simulink model "SimpleStack"  (R2023b)
settings: Solver=ode4  StartTime=0.0  StopTime=10.0  FixedStep=1e-4  RelTol=1e-6
undefined symbols (not defined in the file): A_stack, M_H2O, M_Nmix, M_O2, m_st_Nmix_init, m_st_O2_init, m_st_vp_init, R_Nmix, R_O2, R_vp, V_stack
settings Model: Creator=KOTA-Z  LastModifiedBy=KOTA-Z

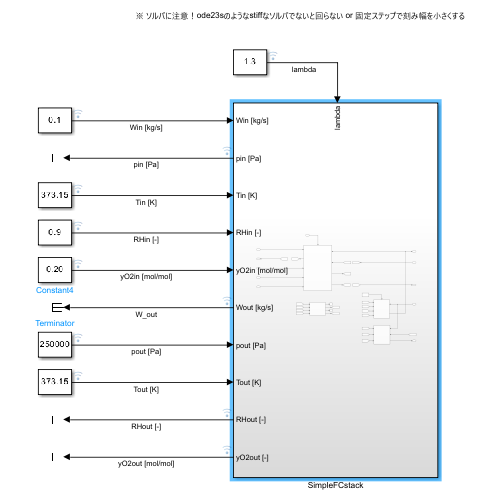
[thumbnail: Simulink's stored preview of the top-level diagram]
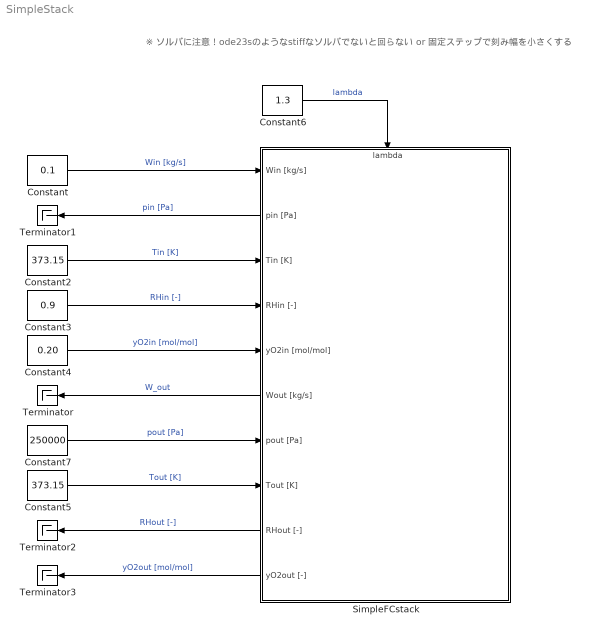
== system SimpleStack ==
  note: ※ ソルバに注意！ode23sのようなstiffなソルバでないと回らない or 固定ステップで刻み幅を小さくする
  Constant : Constant  Value=0.1
  Constant2 : Constant  Value=373.15
  Constant3 : Constant  Value=0.9
  Constant4 : Constant  Value=0.20
  Constant5 : Constant  Value=373.15
  Constant6 : Constant  Value=1.3
  Constant7 : Constant  Value=250000
  SimpleFCstack : Subsystem
      settings: PortSchema="{\"entries\":[{\"content\":{\"sides\":[{\"content\":{\"connectorIds\":[\"In1\",\"Out1\",\"In2\",\"In3\",\"In4\",\"Out2\",\"In5\",\"In6\",\"Out3\",\"Out4\"]},\"type\":\"ConnectorPlacement.EquallySpacedRectSide\",\"uuid\":\"655c3a5c-2438-4b8a-8343-42ad601375b4\"},{\"content\":{\"side\":\"RIGHT\"},\"type\":\"ConnectorPlacement.EquallySpacedRectSide\",\"uuid\":\"d33e9b8c-45a6-4977-af4d-86fbf3e4639a\"},{\"content\":{\"connectorIds\":[\"In7\"],\"side\":\"TOP\"},\"type\":\"ConnectorPlacement.EquallySpacedRectSide\",\"uuid\":\"600fa4b4-34fc-436b-99fc-6adfd4c4a471\"}]},\"type\":\"ConnectorPlacement.EquallySpacedConnector\",\"uuid\":\"963465b0-aa19-4ba1-823c-60c91f5f4c3b\"}],\"packageUris\":[\"http://schema.mathworks.com/mf0/Connector/R2020b\"],\"version\":\"1.0\"}"
  Terminator{,1..3} (4 alike) : Terminator
  wires:
  Constant5/1 -> SimpleFCstack/6(Tout [K])  "Tout [K]"
  Constant4/1 -> SimpleFCstack/4(yO2in [mol/mol])  "yO2in [mol/mol]"
  Constant/1 -> SimpleFCstack/1(Win [kg/s])  "Win [kg/s]"
  Constant3/1 -> SimpleFCstack/3(RHin [-])  "RHin [-]"
  SimpleFCstack/1(pin [Pa]) -> Terminator1/1  "pin [Pa]"
  SimpleFCstack/4(yO2out [-]) -> Terminator3/1  "yO2out [mol/mol]"
  Constant7/1 -> SimpleFCstack/5(pout [Pa])  "pout [Pa]"
  SimpleFCstack/2(Wout [kg/s]) -> Terminator/1  "W_out"
  Constant6/1 -> SimpleFCstack/7(lambda)  "lambda"
  SimpleFCstack/3(RHout [-]) -> Terminator2/1  "RHout [-]"
  Constant2/1 -> SimpleFCstack/2(Tin [K])  "Tin [K]"

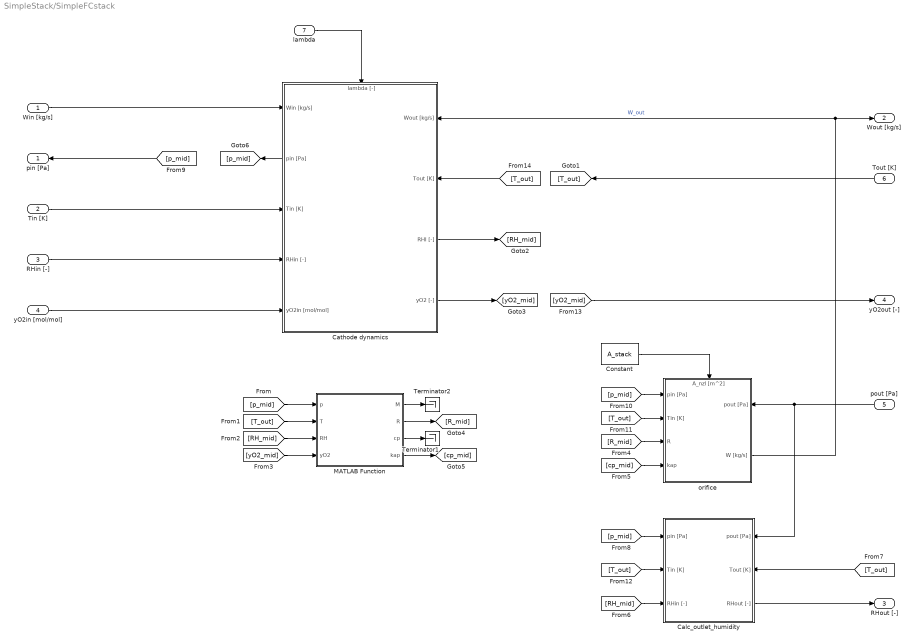
== system SimpleStack/SimpleFCstack ==
  Win [kg/s] : Inport
  Tin [K] : Inport  Port=2
  RHin [-] : Inport  Port=3
  yO2in [mol/mol] : Inport  Port=4
  pout [Pa] : Inport  Port=5
  Tout [K] : Inport  Port=6
  lambda : Inport  Port=7
  Calc_outlet_humidity : Subsystem
      settings: PortSchema="{\"entries\":[{\"content\":{\"sides\":[{\"content\":{\"connectorIds\":[\"In1\",\"In2\",\"In3\"]},\"type\":\"ConnectorPlacement.EquallySpacedRectSide\",\"uuid\":\"71f38106-807e-4ed0-ae6c-bbacb474f6c2\"},{\"content\":{\"connectorIds\":[\"In4\",\"In5\",\"Out1\"],\"side\":\"RIGHT\"},\"type\":\"ConnectorPlacement.EquallySpacedRectSide\",\"uuid\":\"6d4269b2-3333-4431-9298-369e5f90d9a7\"},{\"content\":{\"side\":\"TOP\"},\"type\":\"ConnectorPlacement.EquallySpacedRectSide\",\"uuid\":\"5a9c4429-cecf-425a-a491-b651e9aa4143\"}]},\"type\":\"ConnectorPlacement.EquallySpacedConnector\",\"uuid\":\"39426d6a-7e43-41a2-9c81-324c7c3acccd\"}],\"packageUris\":[\"http://schema.mathworks.com/mf0/Connector/R2020b\"],\"version\":\"1.0\"}"
  Cathode dynamics : Subsystem
      settings: PortSchema="{\"entries\":[{\"content\":{\"sides\":[{\"content\":{\"connectorIds\":[\"In1\",\"Out3\",\"In2\",\"In3\",\"In4\"]},\"type\":\"ConnectorPlacement.EquallySpacedRectSide\",\"uuid\":\"fa7fb944-b3f2-4d7f-acb3-ff4b9695f5bb\"},{\"content\":{\"connectorIds\":[\"In6\",\"In7\",\"Out1\",\"Out2\"],\"side\":\"RIGHT\"},\"type\":\"ConnectorPlacement.EquallySpacedRectSide\",\"uuid\":\"c44f1f17-fb15-4535-ad6a-0eca26be82eb\"},{\"content\":{\"connectorIds\":[\"In5\"],\"side\":\"TOP\"},\"type\":\"ConnectorPlacement.EquallySpacedRectSide\",\"uuid\":\"3976ae6f-6c41-45df-9f2a-11517639fca1\"}]},\"type\":\"ConnectorPlacement.EquallySpacedConnector\",\"uuid\":\"2e8d1e31-2d62-44f7-94c0-4e740688e650\"}],\"packageUris\":[\"http://schema.mathworks.com/mf0/Connector/R2020b\"],\"version\":\"1.0\"}"
  Constant : Constant  Value=A_stack
  MATLAB Function : MATLAB Function  TreatAsAtomicUnit=on  mask{M_O2=M_O2, M_Nmix=M_Nmix, M_H2O=M_H2O}
      mask prompts: M_O2 "Molar mass O2 [kg/mol]"; M_Nmix "Molar mass Nmix [kg/mol]"; M_H2O "Molar mass H2O [kg/mol]"
  Terminator1 : Terminator
  Terminator2 : Terminator
  orifice : Subsystem
      settings: PortSchema="{\"entries\":[{\"content\":{\"sides\":[{\"content\":{\"connectorIds\":[\"In1\",\"In2\",\"In3\",\"In4\"]},\"type\":\"ConnectorPlacement.EquallySpacedRectSide\",\"uuid\":\"efae8970-47c5-4a02-bf2c-57821bb85d37\"},{\"content\":{\"connectorIds\":[\"In6\",\"Out1\"],\"side\":\"RIGHT\"},\"type\":\"ConnectorPlacement.EquallySpacedRectSide\",\"uuid\":\"c072edf9-8db2-4656-9a6c-525b54cf676d\"},{\"content\":{\"connectorIds\":[\"In5\"],\"side\":\"TOP\"},\"type\":\"ConnectorPlacement.EquallySpacedRectSide\",\"uuid\":\"a5f35e53-894b-4e4e-8f09-bf3a2c067244\"},{\"content\":{\"side\":\"BOTTOM\"},\"type\":\"ConnectorPlacement.EquallySpacedRectSide\",\"uuid\":\"c3ea8794-d4c2-446d-854c-4c5a5875e6e6\"}]},\"type\":\"ConnectorPlacement.EquallySpacedConnector\",\"uuid\":\"567c8408-e503-409c-8be3-b925cf408148\"}],\"packageUris\":[\"http://schema.mathworks.com/mf0/Connector/R2020b\"],\"version\":\"1.0\"}"
  pin [Pa] : Outport
  Wout [kg/s] : Outport  Port=2
  RHout [-] : Outport  Port=3
  yO2out [-] : Outport  Port=4
  wires:
  pout [Pa]/1 -> orifice/6(pout [Pa]), Calc_outlet_humidity/4(pout [Pa])
  orifice/1(W [kg/s]) -> Cathode dynamics/6(Wout [kg/s]), Wout [kg/s]/1  "W_out"
  Constant/1 -> orifice/5(A_nzl [m^2])
  Cathode dynamics/2(yO2 [-]) -> [yO2_mid]
  Win [kg/s]/1 -> Cathode dynamics/1(Win [kg/s])
  [p_mid] -> pin [Pa]/1
  lambda/1 -> Cathode dynamics/5(lambda [-])
  Tin [K]/1 -> Cathode dynamics/2(Tin [K])
  RHin [-]/1 -> Cathode dynamics/3(RHin [-])
  yO2in [mol/mol]/1 -> Cathode dynamics/4(yO2in [mol/mol])
  Calc_outlet_humidity/1(RHout [-]) -> RHout [-]/1
  MATLAB Function/1(M) -> Terminator2/1
  MATLAB Function/3(cp) -> Terminator1/1
  Cathode dynamics/1(RHI [-]) -> [RH_mid]
  [p_mid] -> MATLAB Function/1(p)
  [T_out] -> MATLAB Function/2(T)
  [RH_mid] -> MATLAB Function/3(RH)
  [yO2_mid] -> MATLAB Function/4(yO2)
  MATLAB Function/2(R) -> [R_mid]
  [R_mid] -> orifice/3(R)
  MATLAB Function/4(kap) -> [cp_mid]
  [cp_mid] -> orifice/4(kap)
  [RH_mid] -> Calc_outlet_humidity/3(RHin [-])
  [T_out] -> Calc_outlet_humidity/5(Tout [K])
  [p_mid] -> Calc_outlet_humidity/1(pin [Pa])
  Cathode dynamics/3(pin [Pa]) -> [p_mid]
  [p_mid] -> orifice/1(pin [Pa])
  [T_out] -> orifice/2(Tin [K])
  [T_out] -> Calc_outlet_humidity/2(Tin [K])
  [yO2_mid] -> yO2out [-]/1
  [T_out] -> Cathode dynamics/7(Tout [K])
  Tout [K]/1 -> [T_out]

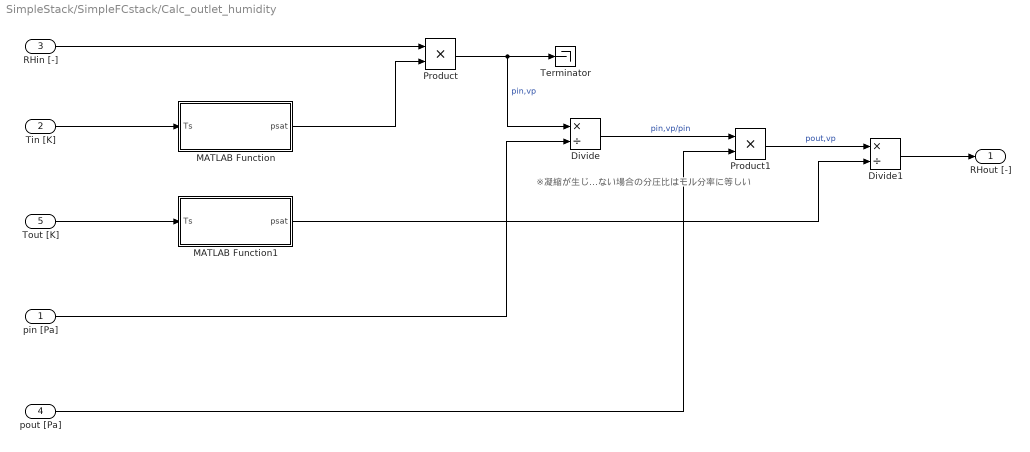
== system SimpleStack/SimpleFCstack/Calc_outlet_humidity ==
  note: ※凝縮が生じない場合の分圧比はモル分率に等しい
  pin [Pa] : Inport
  Tin [K] : Inport  Port=2
  RHin [-] : Inport  Port=3
  pout [Pa] : Inport  Port=4
  Tout [K] : Inport  Port=5
  Divide : Product  Inputs=*/
  Divide1 : Product  Inputs=*/
  MATLAB Function : MATLAB Function  TreatAsAtomicUnit=on
  MATLAB Function1 : MATLAB Function  TreatAsAtomicUnit=on
  Product : Product
  Product1 : Product
  Terminator : Terminator
  RHout [-] : Outport
  wires:
  MATLAB Function/1(psat) -> Product/2
  Tin [K]/1 -> MATLAB Function/1(Ts)
  Tout [K]/1 -> MATLAB Function1/1(Ts)
  RHin [-]/1 -> Product/1
  Product/1 -> Terminator/1, Divide/1  "pin,vp"
  pin [Pa]/1 -> Divide/2
  Divide/1 -> Product1/1  "pin,vp/pin"
  pout [Pa]/1 -> Product1/2
  Product1/1 -> Divide1/1  "pout,vp"
  MATLAB Function1/1(psat) -> Divide1/2
  Divide1/1 -> RHout [-]/1

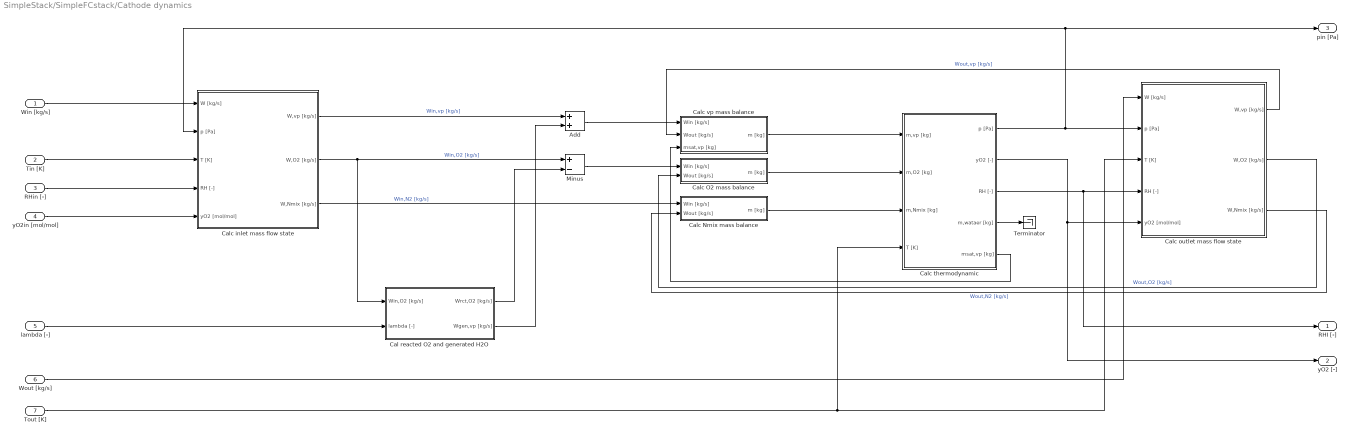
== system SimpleStack/SimpleFCstack/Cathode dynamics ==
  Win [kg/s] : Inport
  Tin [K] : Inport  Port=2
  RHin [-] : Inport  Port=3
  yO2in [mol/mol] : Inport  Port=4
  lambda [-] : Inport  Port=5
  Wout [kg/s] : Inport  Port=6
  Tout [K] : Inport  Port=7
  Add : Sum
  Cal reacted O2 and generated H2O : Subsystem
  Calc Nmix mass balance : Subsystem
  Calc O2 mass balance : Subsystem
  Calc inlet mass flow state : Subsystem
  Calc outlet mass flow state : Subsystem
  Calc thermodynamic : Subsystem
  Calc vp mass balance : Subsystem
  Minus : Sum  Inputs=+-
  Terminator : Terminator
  RHI [-] : Outport
  yO2 [-] : Outport  Port=2
  pin [Pa] : Outport  Port=3
  wires:
  Calc outlet mass flow state/3(W,Nmix [kg/s]) -> Calc Nmix mass balance/2(Wout [kg/s])  "Wout,N2 [kg/s]"
  Calc vp mass balance/1(m [kg]) -> Calc thermodynamic/1(m,vp [kg])
  RHin [-]/1 -> Calc inlet mass flow state/4(RH [-])
  Calc outlet mass flow state/1(W,vp [kg/s]) -> Calc vp mass balance/2(Wout [kg/s])  "Wout,vp [kg/s]"
  Calc inlet mass flow state/2(W,O2 [kg/s]) -> Minus/1, Cal reacted O2 and generated H2O/1(Win,O2 [kg/s])  "Win,O2 [kg/s]"
  Win [kg/s]/1 -> Calc inlet mass flow state/1(W [kg/s])
  Calc O2 mass balance/1(m [kg]) -> Calc thermodynamic/2(m,O2 [kg])
  lambda [-]/1 -> Cal reacted O2 and generated H2O/2(lambda [-])
  Minus/1 -> Calc O2 mass balance/1(Win [kg/s])
  Calc thermodynamic/2(yO2 [-]) -> yO2 [-]/1, Calc outlet mass flow state/5(yO2 [mol/mol])
  Tout [K]/1 -> Calc outlet mass flow state/3(T [K]), Calc thermodynamic/4(T [K])
  Calc outlet mass flow state/2(W,O2 [kg/s]) -> Calc O2 mass balance/2(Wout [kg/s])  "Wout,O2 [kg/s]"
  Calc inlet mass flow state/3(W,Nmix [kg/s]) -> Calc Nmix mass balance/1(Win [kg/s])  "Win,N2 [kg/s]"
  Calc Nmix mass balance/1(m [kg]) -> Calc thermodynamic/3(m,Nmix [kg])
  Calc thermodynamic/3(RH [-]) -> RHI [-]/1, Calc outlet mass flow state/4(RH [-])
  Calc thermodynamic/4(m,wataer [kg]) -> Terminator/1
  Cal reacted O2 and generated H2O/1(Wrct,O2 [kg/s]) -> Minus/2
  Calc thermodynamic/5(msat,vp [kg]) -> Calc vp mass balance/3(msat,vp [kg])
  Tin [K]/1 -> Calc inlet mass flow state/3(T [K])
  Calc inlet mass flow state/1(W,vp [kg/s]) -> Add/1  "Win,vp [kg/s]"
  Add/1 -> Calc vp mass balance/1(Win [kg/s])
  yO2in [mol/mol]/1 -> Calc inlet mass flow state/5(yO2 [mol/mol])
  Cal reacted O2 and generated H2O/2(Wgen,vp [kg/s]) -> Add/2
  Calc thermodynamic/1(p [Pa]) -> pin [Pa]/1, Calc inlet mass flow state/2(p [Pa]), Calc outlet mass flow state/2(p [Pa])
  Wout [kg/s]/1 -> Calc outlet mass flow state/1(W [kg/s])

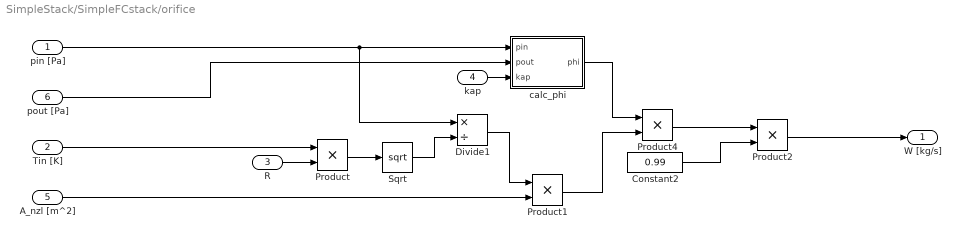
== system SimpleStack/SimpleFCstack/orifice ==
  pin [Pa] : Inport
  Tin [K] : Inport  Port=2
  R : Inport  Port=3
  kap : Inport  Port=4
  A_nzl [m^2] : Inport  Port=5
  pout [Pa] : Inport  Port=6
  Constant2 : Constant  Value=0.99
  Divide1 : Product  Inputs=*/
  Product{,1..2,4} (4 alike) : Product
  Sqrt : Sqrt
  calc_phi : MATLAB Function  TreatAsAtomicUnit=on
  W [kg/s] : Outport
  wires:
  pout [Pa]/1 -> calc_phi/2(pout)
  pin [Pa]/1 -> calc_phi/1(pin), Divide1/1
  Tin [K]/1 -> Product/1
  A_nzl [m^2]/1 -> Product1/2
  R/1 -> Product/2
  Product/1 -> Sqrt/1
  Sqrt/1 -> Divide1/2
  Divide1/1 -> Product1/1
  kap/1 -> calc_phi/3(kap)
  calc_phi/1(phi) -> Product4/1
  Product1/1 -> Product4/2
  Product4/1 -> Product2/1
  Product2/1 -> W [kg/s]/1
  Constant2/1 -> Product2/2

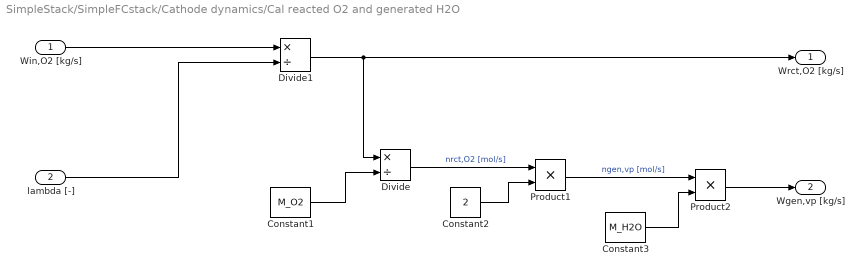
== system SimpleStack/SimpleFCstack/Cathode dynamics/Cal reacted O2 and generated H2O ==
  Win,O2 [kg/s] : Inport
  lambda [-] : Inport  Port=2
  Constant1 : Constant  Value=M_O2
  Constant2 : Constant  Value=2
  Constant3 : Constant  Value=M_H2O
  Divide : Product  Inputs=*/
  Divide1 : Product  Inputs=*/  RndMeth=Zero  SaturateOnIntegerOverflow=on
  Product1 : Product
  Product2 : Product
  Wrct,O2 [kg/s] : Outport
  Wgen,vp [kg/s] : Outport  Port=2
  wires:
  Divide1/1 -> Wrct,O2 [kg/s]/1, Divide/1
  Win,O2 [kg/s]/1 -> Divide1/1
  Constant1/1 -> Divide/2
  Divide/1 -> Product1/1  "nrct,O2 [mol/s]"
  Constant2/1 -> Product1/2
  Product1/1 -> Product2/1  "ngen,vp [mol/s]"
  Constant3/1 -> Product2/2
  Product2/1 -> Wgen,vp [kg/s]/1
  lambda [-]/1 -> Divide1/2

== system SimpleStack/SimpleFCstack/Cathode dynamics/Calc Nmix mass balance ==
  Win [kg/s] : Inport
  Wout [kg/s] : Inport  Port=2
  Integrator : Integrator  InitialCondition=m_st_Nmix_init
  Minus : Sum  Inputs=+-
  m [kg] : Outport
  wires:
  Win [kg/s]/1 -> Minus/1
  Wout [kg/s]/1 -> Minus/2
  Minus/1 -> Integrator/1
  Integrator/1 -> m [kg]/1

== system SimpleStack/SimpleFCstack/Cathode dynamics/Calc O2 mass balance ==
  Win [kg/s] : Inport
  Wout [kg/s] : Inport  Port=2
  Integrator : Integrator  InitialCondition=m_st_O2_init
  Minus : Sum  Inputs=+-
  m [kg] : Outport
  wires:
  Integrator/1 -> m [kg]/1
  Minus/1 -> Integrator/1
  Wout [kg/s]/1 -> Minus/2
  Win [kg/s]/1 -> Minus/1

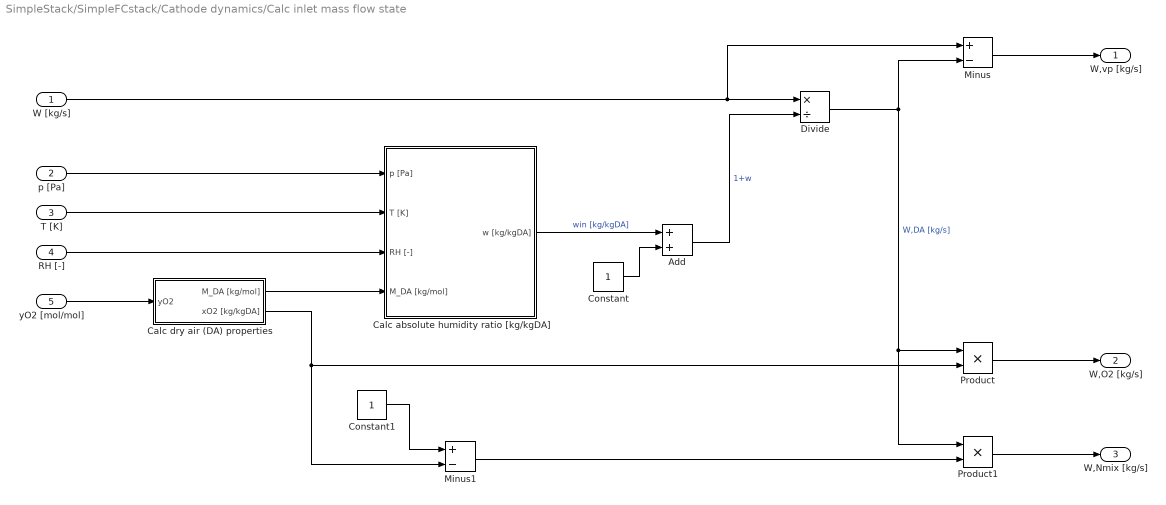
== system SimpleStack/SimpleFCstack/Cathode dynamics/Calc inlet mass flow state ==
  W [kg/s] : Inport
  p [Pa] : Inport  Port=2
  T [K] : Inport  Port=3
  RH [-] : Inport  Port=4
  yO2 [mol/mol] : Inport  Port=5
  Add : Sum
  Calc absolute humidity ratio [kg/kgDA] : Subsystem
  Calc dry air (DA) properties : Subsystem
  Constant : Constant
  Constant1 : Constant
  Divide : Product  Inputs=*/
  Minus : Sum  Inputs=+-
  Minus1 : Sum  Inputs=+-
  Product : Product
  Product1 : Product
  W,vp [kg/s] : Outport
  W,O2 [kg/s] : Outport  Port=2
  W,Nmix [kg/s] : Outport  Port=3
  wires:
  p [Pa]/1 -> Calc absolute humidity ratio [kg/kgDA]/1(p [Pa])
  Calc dry air (DA) properties/2(xO2 [kg/kgDA]) -> Minus1/2, Product/2
  Calc absolute humidity ratio [kg/kgDA]/1(w [kg/kgDA]) -> Add/1  "win [kg/kgDA]"
  Calc dry air (DA) properties/1(M_DA [kg/mol]) -> Calc absolute humidity ratio [kg/kgDA]/4(M_DA [kg/mol])
  Product/1 -> W,O2 [kg/s]/1
  Divide/1 -> Minus/2, Product1/1, Product/1  "W,DA [kg/s]"
  Product1/1 -> W,Nmix [kg/s]/1
  Minus1/1 -> Product1/2
  Minus/1 -> W,vp [kg/s]/1
  yO2 [mol/mol]/1 -> Calc dry air (DA) properties/1(yO2)
  Constant1/1 -> Minus1/1
  RH [-]/1 -> Calc absolute humidity ratio [kg/kgDA]/3(RH [-])
  W [kg/s]/1 -> Minus/1, Divide/1
  Constant/1 -> Add/2
  Add/1 -> Divide/2  "1+w"
  T [K]/1 -> Calc absolute humidity ratio [kg/kgDA]/2(T [K])

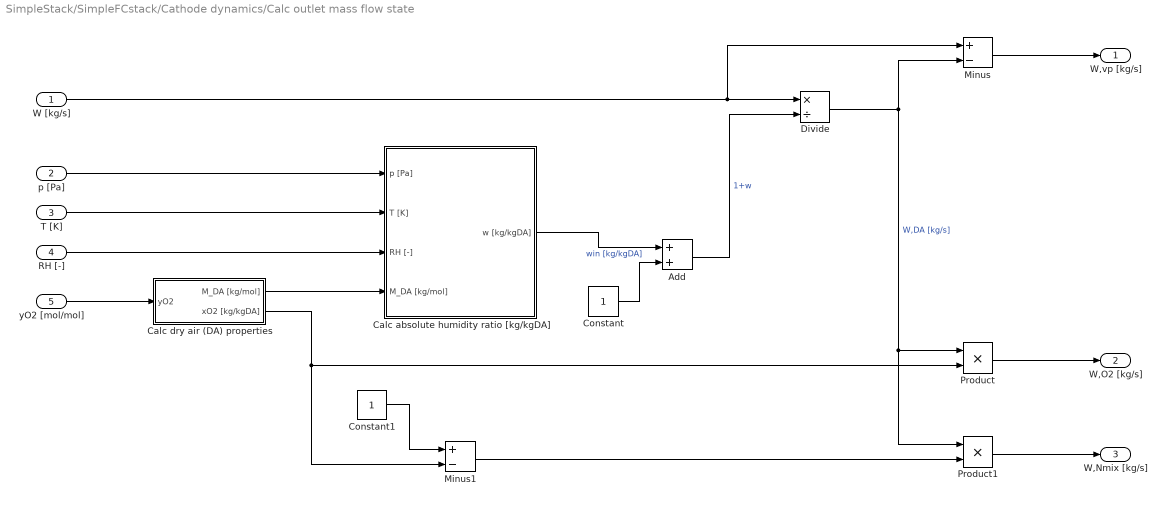
== system SimpleStack/SimpleFCstack/Cathode dynamics/Calc outlet mass flow state ==
  W [kg/s] : Inport
  p [Pa] : Inport  Port=2
  T [K] : Inport  Port=3
  RH [-] : Inport  Port=4
  yO2 [mol/mol] : Inport  Port=5
  Add : Sum
  Calc absolute humidity ratio [kg/kgDA] : Subsystem
  Calc dry air (DA) properties : Subsystem
  Constant : Constant
  Constant1 : Constant
  Divide : Product  Inputs=*/
  Minus : Sum  Inputs=+-
  Minus1 : Sum  Inputs=+-
  Product : Product
  Product1 : Product
  W,vp [kg/s] : Outport
  W,O2 [kg/s] : Outport  Port=2
  W,Nmix [kg/s] : Outport  Port=3
  wires:
  T [K]/1 -> Calc absolute humidity ratio [kg/kgDA]/2(T [K])
  Add/1 -> Divide/2  "1+w"
  Constant/1 -> Add/2
  W [kg/s]/1 -> Divide/1, Minus/1
  RH [-]/1 -> Calc absolute humidity ratio [kg/kgDA]/3(RH [-])
  Constant1/1 -> Minus1/1
  yO2 [mol/mol]/1 -> Calc dry air (DA) properties/1(yO2)
  Minus/1 -> W,vp [kg/s]/1
  Minus1/1 -> Product1/2
  Product1/1 -> W,Nmix [kg/s]/1
  Divide/1 -> Product/1, Product1/1, Minus/2  "W,DA [kg/s]"
  Product/1 -> W,O2 [kg/s]/1
  Calc dry air (DA) properties/1(M_DA [kg/mol]) -> Calc absolute humidity ratio [kg/kgDA]/4(M_DA [kg/mol])
  Calc absolute humidity ratio [kg/kgDA]/1(w [kg/kgDA]) -> Add/1  "win [kg/kgDA]"
  Calc dry air (DA) properties/2(xO2 [kg/kgDA]) -> Minus1/2, Product/2
  p [Pa]/1 -> Calc absolute humidity ratio [kg/kgDA]/1(p [Pa])

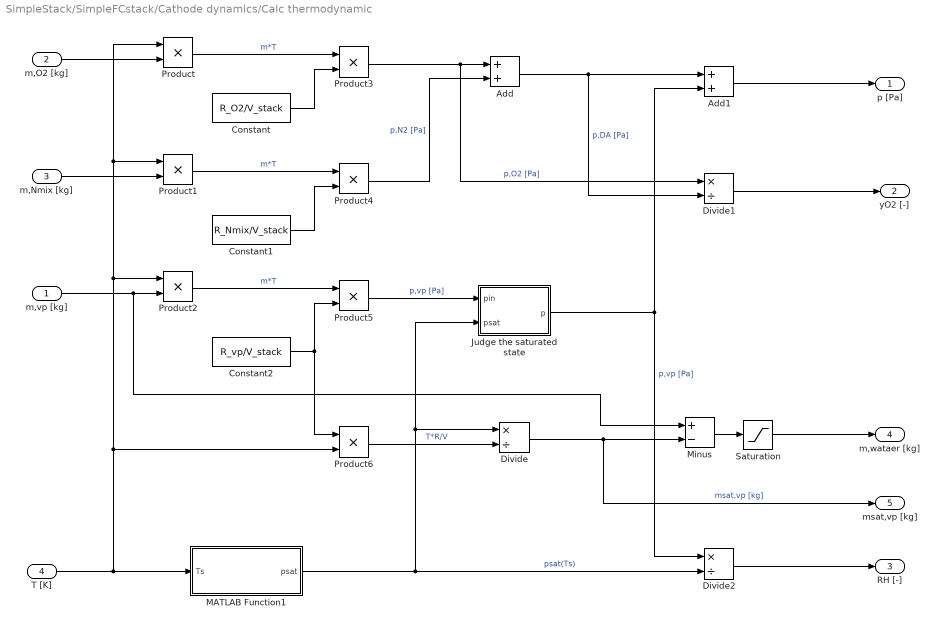
== system SimpleStack/SimpleFCstack/Cathode dynamics/Calc thermodynamic ==
  m,vp [kg] : Inport
  m,O2 [kg] : Inport  Port=2
  m,Nmix [kg] : Inport  Port=3
  T [K] : Inport  Port=4
  Add : Sum
  Add1 : Sum
  Constant : Constant  Value=R_O2/V_stack
  Constant1 : Constant  Value=R_Nmix/V_stack
  Constant2 : Constant  Value=R_vp/V_stack
  Divide : Product  Inputs=*/
  Divide1 : Product  Inputs=*/
  Divide2 : Product  Inputs=*/
  Judge the saturated state : MATLAB Function  TreatAsAtomicUnit=on
  MATLAB Function1 : MATLAB Function  TreatAsAtomicUnit=on
  Minus : Sum  Inputs=+-
  Product{,1..6} (7 alike) : Product
  Saturation : Saturate  UpperLimit=inf  LowerLimit=0
  p [Pa] : Outport
  yO2 [-] : Outport  Port=2
  RH [-] : Outport  Port=3
  m,wataer [kg] : Outport  Port=4
  msat,vp [kg] : Outport  Port=5
  wires:
  m,O2 [kg]/1 -> Product/2
  m,Nmix [kg]/1 -> Product1/2
  m,vp [kg]/1 -> Minus/1, Product2/2
  T [K]/1 -> MATLAB Function1/1(Ts), Product2/1, Product1/1, Product/1, Product6/2
  Product/1 -> Product3/1  "m*T"
  Product1/1 -> Product4/1  "m*T"
  Product2/1 -> Product5/1  "m*T"
  Constant/1 -> Product3/2
  Constant1/1 -> Product4/2
  Constant2/1 -> Product6/1, Product5/2
  Product5/1 -> Judge the saturated state/1(pin)  "p,vp [Pa]"
  MATLAB Function1/1(psat) -> Divide2/2, Divide/1, Judge the saturated state/2(psat)  "psat(Ts)"
  Product6/1 -> Divide/2  "T*R/V"
  Divide/1 -> msat,vp [kg]/1, Minus/2  "msat,vp [kg]"
  Product3/1 -> Divide1/1, Add/1  "p,O2 [Pa]"
  Product4/1 -> Add/2  "p,N2 [Pa]"
  Add/1 -> Add1/1, Divide1/2  "p,DA [Pa]"
  Divide1/1 -> yO2 [-]/1
  Add1/1 -> p [Pa]/1
  Judge the saturated state/1(p) -> Add1/2, Divide2/1  "p,vp [Pa]"
  Minus/1 -> Saturation/1
  Saturation/1 -> m,wataer [kg]/1
  Divide2/1 -> RH [-]/1

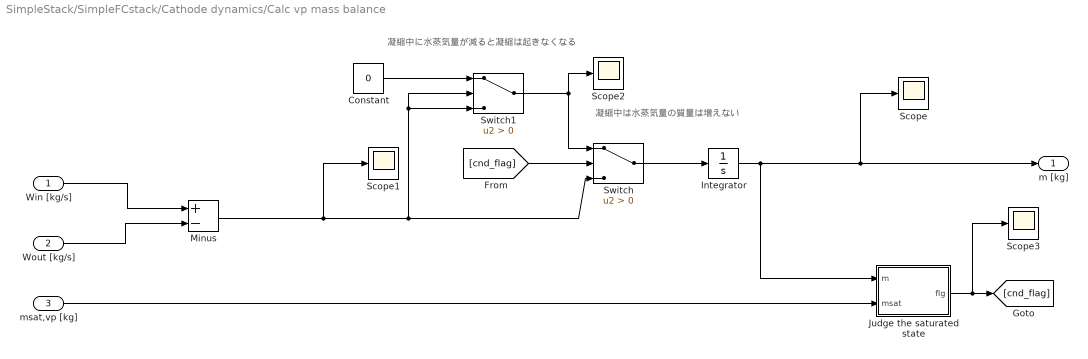
== system SimpleStack/SimpleFCstack/Cathode dynamics/Calc vp mass balance ==
  note: 凝縮中は水蒸気量の質量は増えない
  note: 凝縮中に水蒸気量が減ると凝縮は起きなくなる
  Win [kg/s] : Inport
  Wout [kg/s] : Inport  Port=2
  msat,vp [kg] : Inport  Port=3
  Constant : Constant  Value=0
  Integrator : Integrator  InitialCondition=m_st_vp_init
  Judge the saturated state : MATLAB Function  TreatAsAtomicUnit=on
  Minus : Sum  Inputs=+-
  Scope{,1..3} (4 alike) : Scope
  Switch : Switch  Criteria=u2 > Threshold  SaturateOnIntegerOverflow=off  InputSameDT=off
  Switch1 : Switch  Criteria=u2 > Threshold  SaturateOnIntegerOverflow=off  InputSameDT=off
  m [kg] : Outport
  wires:
  Win [kg/s]/1 -> Minus/1
  Wout [kg/s]/1 -> Minus/2
  [cnd_flag] -> Switch/2
  Minus/1 -> Scope1/1, Switch1/2, Switch1/3, Switch/3
  Switch/1 -> Integrator/1
  Integrator/1 -> Judge the saturated state/1(m), Scope/1, m [kg]/1
  msat,vp [kg]/1 -> Judge the saturated state/2(msat)
  Constant/1 -> Switch1/1
  Judge the saturated state/1(flg) -> Scope3/1, [cnd_flag]
  Switch1/1 -> Switch/1, Scope2/1

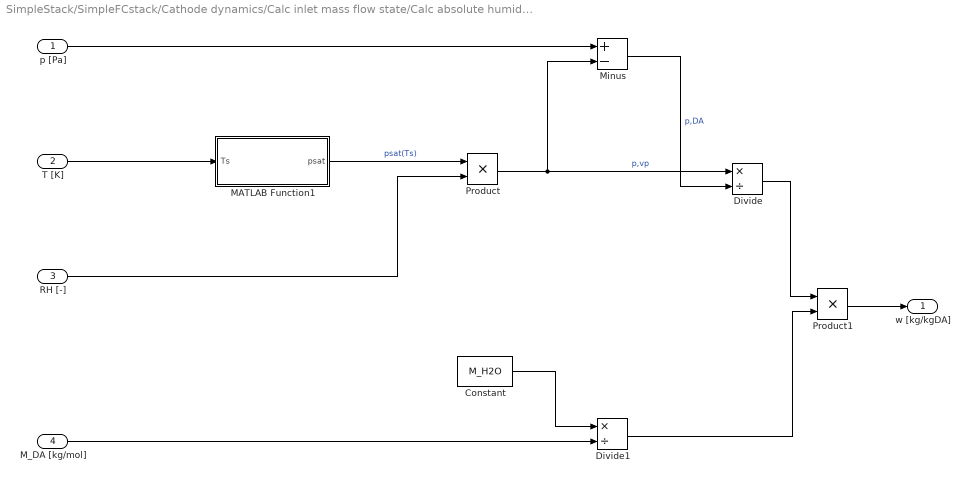
== system SimpleStack/SimpleFCstack/Cathode dynamics/Calc inlet mass flow state/Calc absolute humidity ratio [kg//kgDA] ==
  p [Pa] : Inport
  T [K] : Inport  Port=2
  RH [-] : Inport  Port=3
  M_DA [kg/mol] : Inport  Port=4
  Constant : Constant  Value=M_H2O
  Divide : Product  Inputs=*/
  Divide1 : Product  Inputs=*/
  MATLAB Function1 : MATLAB Function  TreatAsAtomicUnit=on
  Minus : Sum  Inputs=+-
  Product : Product
  Product1 : Product
  w [kg/kgDA] : Outport
  wires:
  T [K]/1 -> MATLAB Function1/1(Ts)
  Minus/1 -> Divide/2  "p,DA"
  Product/1 -> Divide/1, Minus/2  "p,vp"
  Divide1/1 -> Product1/2
  RH [-]/1 -> Product/2
  M_DA [kg/mol]/1 -> Divide1/2
  Constant/1 -> Divide1/1
  Product1/1 -> w [kg/kgDA]/1
  MATLAB Function1/1(psat) -> Product/1  "psat(Ts)"
  Divide/1 -> Product1/1
  p [Pa]/1 -> Minus/1

== system SimpleStack/SimpleFCstack/Cathode dynamics/Calc inlet mass flow state/Calc dry air (DA) properties ==
  yO2 : Inport
  Add1 : Sum
  Constant1 : Constant  Value=M_O2
  Constant2 : Constant
  Constant3 : Constant  Value=M_Nmix
  Divide : Product  Inputs=*/
  Minus : Sum  Inputs=+-
  Product : Product
  Product1 : Product
  M_DA [kg/mol] : Outport
  xO2 [kg/kgDA] : Outport  Port=2
  wires:
  Product/1 -> Divide/1, Add1/1  "m_O2 [kg/molDA]"
  Constant2/1 -> Minus/1
  Constant3/1 -> Product1/1
  Minus/1 -> Product1/2  "1-yO2"
  yO2/1 -> Minus/2, Product/2
  Add1/1 -> M_DA [kg/mol]/1, Divide/2  "M_DA [kg/mol]"
  Constant1/1 -> Product/1
  Product1/1 -> Add1/2
  Divide/1 -> xO2 [kg/kgDA]/1

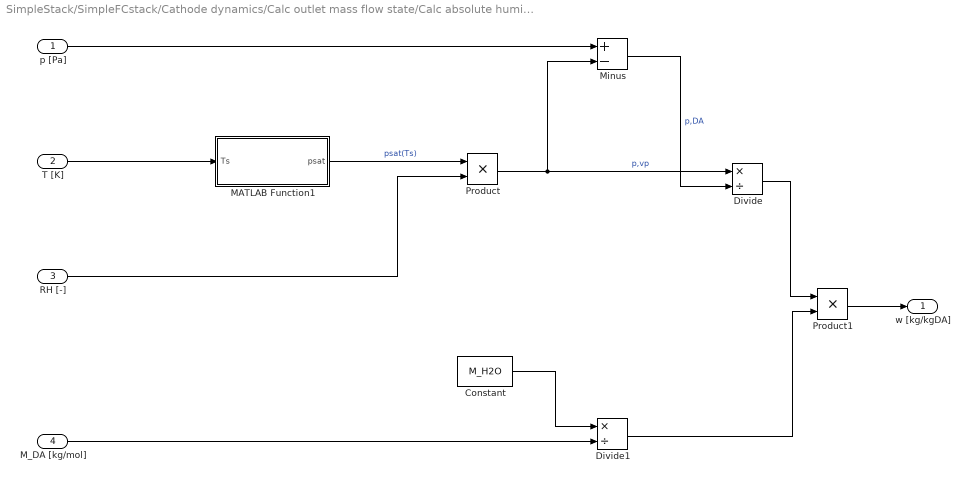
== system SimpleStack/SimpleFCstack/Cathode dynamics/Calc outlet mass flow state/Calc absolute humidity ratio [kg//kgDA] ==
  p [Pa] : Inport
  T [K] : Inport  Port=2
  RH [-] : Inport  Port=3
  M_DA [kg/mol] : Inport  Port=4
  Constant : Constant  Value=M_H2O
  Divide : Product  Inputs=*/
  Divide1 : Product  Inputs=*/
  MATLAB Function1 : MATLAB Function  TreatAsAtomicUnit=on
  Minus : Sum  Inputs=+-
  Product : Product
  Product1 : Product
  w [kg/kgDA] : Outport
  wires:
  p [Pa]/1 -> Minus/1
  Divide/1 -> Product1/1
  MATLAB Function1/1(psat) -> Product/1  "psat(Ts)"
  Product1/1 -> w [kg/kgDA]/1
  Constant/1 -> Divide1/1
  M_DA [kg/mol]/1 -> Divide1/2
  RH [-]/1 -> Product/2
  Divide1/1 -> Product1/2
  Product/1 -> Minus/2, Divide/1  "p,vp"
  Minus/1 -> Divide/2  "p,DA"
  T [K]/1 -> MATLAB Function1/1(Ts)

== system SimpleStack/SimpleFCstack/Cathode dynamics/Calc outlet mass flow state/Calc dry air (DA) properties ==
  yO2 : Inport
  Add1 : Sum
  Constant1 : Constant  Value=M_O2
  Constant2 : Constant
  Constant3 : Constant  Value=M_Nmix
  Divide : Product  Inputs=*/
  Minus : Sum  Inputs=+-
  Product : Product
  Product1 : Product
  M_DA [kg/mol] : Outport
  xO2 [kg/kgDA] : Outport  Port=2
  wires:
  Divide/1 -> xO2 [kg/kgDA]/1
  Product1/1 -> Add1/2
  Constant1/1 -> Product/1
  Add1/1 -> Divide/2, M_DA [kg/mol]/1  "M_DA [kg/mol]"
  yO2/1 -> Product/2, Minus/2
  Minus/1 -> Product1/2  "1-yO2"
  Constant3/1 -> Product1/1
  Constant2/1 -> Minus/1
  Product/1 -> Add1/1, Divide/1  "m_O2 [kg/molDA]"

== matlab function SimpleStack/SimpleFCstack/Cathode dynamics/Calc inlet mass flow state/Calc absolute humidity ratio [kg//kgDA]/MATLAB Function1 ==
  data: Ts input; psat output
function psat = sat_vp_pressure(Ts)
    P_CONVERT = 0.001;
    C1 = -5.6745359e3;
    C2 = 6.3925247;
    C3 = -9.6778430e-3;
    C4 = 6.2215701e-7;
    C5 = 2.0747825e-9;
    C6 = -9.4840240e-13;
    C7 = 4.1635019;
    N1 = 0.11670521452767e4;
    N2 = -0.72421316703206e6;
    N3 = -0.17073846940092e2;
    N4 = 0.12020824702470e5;
    N5 = -0.32325550322333e7;
    N6 = 0.14915108613530e2;
    N7 = -0.4823265731591e4;
    N8 = 0.40511340542057e6;
    N9 = -0.23855557567849e0;
    N10 = 0.65017534844798e3;
    
    if Ts < 273.15+0.01
        % -100~0.01C//三重点を計算以下は wexler-hyland のシミュレーションプログラム式
        psat = exp(C1 / Ts + C2 + C3 * Ts + C4 * Ts^2 + C5 * Ts^3 + C6 * Ts^4 + C7 * log(Ts)) * P_CONVERT;
    else
        %　~647.096K//臨界温度まで一定とするは IAPWS-IF97 実用国際状態式
        alpha = Ts + N9 / (Ts - N10);
        a2 = alpha * alpha;
        A = a2 + N1 * alpha + N2;
        B = N3 * a2 + N4 * alpha + N5;
        C = N6 * a2 + N7 * alpha + N8;
        psat = (2 * C / (-B + (B * B - 4 * A * C)^0.5))^4 / P_CONVERT;
    end 
    psat = psat*1000; %kPa to Pa
end

== matlab function SimpleStack/SimpleFCstack/Cathode dynamics/Calc outlet mass flow state/Calc absolute humidity ratio [kg//kgDA]/MATLAB Function1 ==
  data: Ts input; psat output
function psat = sat_vp_pressure(Ts)
    P_CONVERT = 0.001;
    C1 = -5.6745359e3;
    C2 = 6.3925247;
    C3 = -9.6778430e-3;
    C4 = 6.2215701e-7;
    C5 = 2.0747825e-9;
    C6 = -9.4840240e-13;
    C7 = 4.1635019;
    N1 = 0.11670521452767e4;
    N2 = -0.72421316703206e6;
    N3 = -0.17073846940092e2;
    N4 = 0.12020824702470e5;
    N5 = -0.32325550322333e7;
    N6 = 0.14915108613530e2;
    N7 = -0.4823265731591e4;
    N8 = 0.40511340542057e6;
    N9 = -0.23855557567849e0;
    N10 = 0.65017534844798e3;
    
    if Ts < 273.15+0.01
        % -100~0.01C//三重点を計算以下は wexler-hyland のシミュレーションプログラム式
        psat = exp(C1 / Ts + C2 + C3 * Ts + C4 * Ts^2 + C5 * Ts^3 + C6 * Ts^4 + C7 * log(Ts)) * P_CONVERT;
    else
        %　~647.096K//臨界温度まで一定とするは IAPWS-IF97 実用国際状態式
        alpha = Ts + N9 / (Ts - N10);
        a2 = alpha * alpha;
        A = a2 + N1 * alpha + N2;
        B = N3 * a2 + N4 * alpha + N5;
        C = N6 * a2 + N7 * alpha + N8;
        psat = (2 * C / (-B + (B * B - 4 * A * C)^0.5))^4 / P_CONVERT;
    end 
    psat = psat*1000; %kPa to Pa
end

== matlab function SimpleStack/SimpleFCstack/Cathode dynamics/Calc thermodynamic/Judge the saturated state ==
  data: pin input; p output; psat input
function p = fcn(pin,psat)
    if pin < psat
        p = pin;
    else
        p = psat;  
    end
end

== matlab function SimpleStack/SimpleFCstack/Cathode dynamics/Calc thermodynamic/MATLAB Function1 ==
  data: Ts input; psat output
function psat = sat_vp_pressure(Ts)
    P_CONVERT = 0.001;
    C1 = -5.6745359e3;
    C2 = 6.3925247;
    C3 = -9.6778430e-3;
    C4 = 6.2215701e-7;
    C5 = 2.0747825e-9;
    C6 = -9.4840240e-13;
    C7 = 4.1635019;
    N1 = 0.11670521452767e4;
    N2 = -0.72421316703206e6;
    N3 = -0.17073846940092e2;
    N4 = 0.12020824702470e5;
    N5 = -0.32325550322333e7;
    N6 = 0.14915108613530e2;
    N7 = -0.4823265731591e4;
    N8 = 0.40511340542057e6;
    N9 = -0.23855557567849e0;
    N10 = 0.65017534844798e3;
    
    if Ts < 273.15+0.01
        % -100~0.01C//三重点を計算以下は wexler-hyland のシミュレーションプログラム式
        psat = exp(C1 / Ts + C2 + C3 * Ts + C4 * Ts^2 + C5 * Ts^3 + C6 * Ts^4 + C7 * log(Ts)) * P_CONVERT;
    else
        %　~647.096K//臨界温度まで一定とするは IAPWS-IF97 実用国際状態式
        alpha = Ts + N9 / (Ts - N10);
        a2 = alpha * alpha;
        A = a2 + N1 * alpha + N2;
        B = N3 * a2 + N4 * alpha + N5;
        C = N6 * a2 + N7 * alpha + N8;
        psat = (2 * C / (-B + (B * B - 4 * A * C)^0.5))^4 / P_CONVERT;
    end 
    psat = psat*1000; %kPa to Pa
end

== matlab function SimpleStack/SimpleFCstack/Cathode dynamics/Calc vp mass balance/Judge the saturated state ==
  data: m input; flg output; msat input
function flg = fcn(m,msat)
    if m < msat
        flg = 0;
    else
        flg = 1;  
    end
end

== matlab function SimpleStack/SimpleFCstack/MATLAB Function ==
  data: p input; T input; RH input; yO2 input; M output; R output; cp output; kap output; M_Nmix parameter; M_H2O parameter; M_O2 parameter
%% 湿り空気の状態量計算
function [M, R, cp, kap] = calc_MA_property(p, T, RH, yO2, M_Nmix, M_H2O, M_O2)
    % 湿り空気の物性値計算
    gsprop = GasProperties;
    [M,R,cp,kap] = gsprop.getMAprop(p, T, RH, yO2);
end

%% Calculate saturated vapor pressure [Pa]
function psat = sat_vp_pressure(Ts)
    P_CONVERT = 0.001;
    C1 = -5.6745359e3;
    C2 = 6.3925247;
    C3 = -9.6778430e-3;
    C4 = 6.2215701e-7;
    C5 = 2.0747825e-9;
    C6 = -9.4840240e-13;
    C7 = 4.1635019;
    N1 = 0.11670521452767e4;
    N2 = -0.72421316703206e6;
    N3 = -0.17073846940092e2;
    N4 = 0.12020824702470e5;
    N5 = -0.32325550322333e7;
    N6 = 0.14915108613530e2;
    N7 = -0.4823265731591e4;
    N8 = 0.40511340542057e6;
    N9 = -0.23855557567849e0;
    N10 = 0.65017534844798e3;
    
    if Ts < 273.15+0.01
        % -100~0.01C//三重点を計算以下は wexler-hyland のシミュレーションプログラム式
        psat = exp(C1 / Ts + C2 + C3 * Ts + C4 * Ts^2 + C5 * Ts^3 + C6 * Ts^4 + C7 * log(Ts)) * P_CONVERT;
    else
        %　~647.096K//臨界温度まで一定とするは IAPWS-IF97 実用国際状態式
        alpha = Ts + N9 / (Ts - N10);
        a2 = alpha * alpha;
        A = a2 + N1 * alpha + N2;
        B = N3 * a2 + N4 * alpha + N5;
        C = N6 * a2 + N7 * alpha + N8;
        psat = (2 * C / (-B + (B * B - 4 * A * C)^0.5))^4 / P_CONVERT;
    end 
    psat = psat*1000; %kPa to Pa
end

== matlab function SimpleStack/SimpleFCstack/Calc_outlet_humidity/MATLAB Function ==
  data: Ts input; psat output
function psat = sat_vp_pressure(Ts)
    P_CONVERT = 0.001;
    C1 = -5.6745359e3;
    C2 = 6.3925247;
    C3 = -9.6778430e-3;
    C4 = 6.2215701e-7;
    C5 = 2.0747825e-9;
    C6 = -9.4840240e-13;
    C7 = 4.1635019;
    N1 = 0.11670521452767e4;
    N2 = -0.72421316703206e6;
    N3 = -0.17073846940092e2;
    N4 = 0.12020824702470e5;
    N5 = -0.32325550322333e7;
    N6 = 0.14915108613530e2;
    N7 = -0.4823265731591e4;
    N8 = 0.40511340542057e6;
    N9 = -0.23855557567849e0;
    N10 = 0.65017534844798e3;
    
    if Ts < 273.15+0.01
        % -100~0.01C//三重点を計算以下は wexler-hyland のシミュレーションプログラム式
        psat = exp(C1 / Ts + C2 + C3 * Ts + C4 * Ts^2 + C5 * Ts^3 + C6 * Ts^4 + C7 * log(Ts)) * P_CONVERT;
    else
        %　~647.096K//臨界温度まで一定とするは IAPWS-IF97 実用国際状態式
        alpha = Ts + N9 / (Ts - N10);
        a2 = alpha * alpha;
        A = a2 + N1 * alpha + N2;
        B = N3 * a2 + N4 * alpha + N5;
        C = N6 * a2 + N7 * alpha + N8;
        psat = (2 * C / (-B + (B * B - 4 * A * C)^0.5))^4 / P_CONVERT;
    end 
    psat = psat*1000; %kPa to Pa
end

== matlab function SimpleStack/SimpleFCstack/Calc_outlet_humidity/MATLAB Function1 ==
  data: Ts input; psat output
function psat = sat_vp_pressure(Ts)
    P_CONVERT = 0.001;
    C1 = -5.6745359e3;
    C2 = 6.3925247;
    C3 = -9.6778430e-3;
    C4 = 6.2215701e-7;
    C5 = 2.0747825e-9;
    C6 = -9.4840240e-13;
    C7 = 4.1635019;
    N1 = 0.11670521452767e4;
    N2 = -0.72421316703206e6;
    N3 = -0.17073846940092e2;
    N4 = 0.12020824702470e5;
    N5 = -0.32325550322333e7;
    N6 = 0.14915108613530e2;
    N7 = -0.4823265731591e4;
    N8 = 0.40511340542057e6;
    N9 = -0.23855557567849e0;
    N10 = 0.65017534844798e3;
    
    if Ts < 273.15+0.01
        % -100~0.01C//三重点を計算以下は wexler-hyland のシミュレーションプログラム式
        psat = exp(C1 / Ts + C2 + C3 * Ts + C4 * Ts^2 + C5 * Ts^3 + C6 * Ts^4 + C7 * log(Ts)) * P_CONVERT;
    else
        %　~647.096K//臨界温度まで一定とするは IAPWS-IF97 実用国際状態式
        alpha = Ts + N9 / (Ts - N10);
        a2 = alpha * alpha;
        A = a2 + N1 * alpha + N2;
        B = N3 * a2 + N4 * alpha + N5;
        C = N6 * a2 + N7 * alpha + N8;
        psat = (2 * C / (-B + (B * B - 4 * A * C)^0.5))^4 / P_CONVERT;
    end 
    psat = psat*1000; %kPa to Pa
end

== matlab function SimpleStack/SimpleFCstack/orifice/calc_phi ==
  data: pin input; phi output; pout input; kap input
function phi = fcn(pin,pout,kap)
    pr = pout/pin;
    p_cr = (2/(kap+1))^(kap/(kap-1))*pin;
    % Judge critical pressure
    if pout < p_cr
        tmp_phi = sqrt(kap*(2/(kap+1))^((kap+1)/(kap-1)));
    else
        % Prevent to become minus values
        a = 1-pr^((kap-1)/kap);
        if a < 0
           a = 0;
        end
        tmp_phi = pr^(1/kap)*sqrt(2*kap/(kap-1)*(a));
    end
    phi = tmp_phi;
end
